simulink model "p1_and_p2_transfer"  (R2025b)
settings: Solver=VariableStepAuto  StartTime=0.0  StopTime=5  RelTol=1e-3
values from neighbouring files (symbols this model uses):
  b = 0.028    [script_p1_to_p4.m]
  J = 0.0113    [script_p1_to_p4.m]
  Ke = 0.067    [script_p1_to_p4.m]
  Kt = 0.067    [script_p1_to_p4.m]
  L = 0.1    [script_p1_to_p4.m]
  R = 0.45    [script_p1_to_p4.m]
settings Model: Creator=Kittitouch Tantiwong  LastModifiedBy=Kittitouch Tantiwong

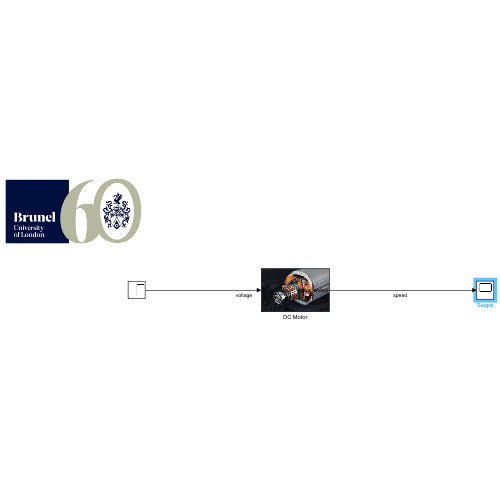
[thumbnail: Simulink's stored preview of the top-level diagram]
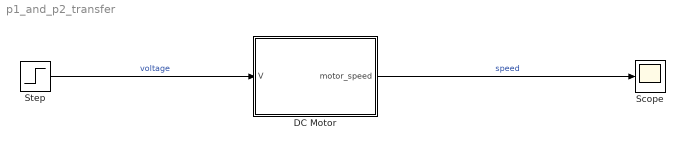
== system p1_and_p2_transfer ==
  DC Motor : Subsystem
      mask Display: image('DC motor.jpg');
  Scope : Scope
      settings: ActiveDisplayYMinimum=-0.49090533490817989  ActiveDisplayYMaximum=4.41814801417362
  Step : Step  SampleTime=0
  wires:
  DC Motor/1(motor_speed) -> Scope/1  "speed"
  Step/1 -> DC Motor/1(V)  "voltage"

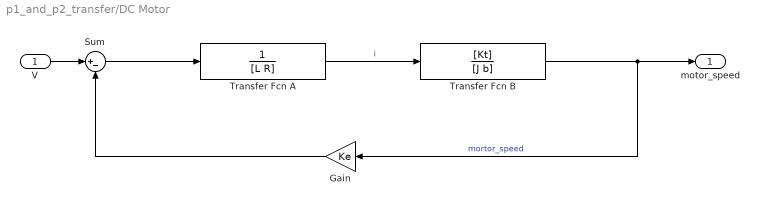
== system p1_and_p2_transfer/DC Motor ==
  V : Inport
  Gain : Gain  Gain=Ke
  Sum : Sum  Inputs=|+-
  Transfer Fcn A : TransferFcn  Denominator=[L R]
  Transfer Fcn B : TransferFcn  Numerator=[Kt]  Denominator=[J b]
  motor_speed : Outport
  wires:
  Transfer Fcn B/1 -> motor_speed/1, Gain/1  "mortor_speed"
  Transfer Fcn A/1 -> Transfer Fcn B/1  "i"
  Sum/1 -> Transfer Fcn A/1
  Gain/1 -> Sum/2
  V/1 -> Sum/1
